simulink model "wtd_wind_profile_ver1"  (R2014b)
settings: Solver=ode3  StartTime=0.0  StopTime=100  FixedStep=0.002  RelTol=1e-3
undefined symbols (not defined in the file): baseSystemPower, complexPower, internalGenVoltage, nodeVoltage, systemFrequency, windSpeedVec, windturbKbParam
libraries: wtd_library_ver1 x11, simulink x1
settings Model: Creator=Jakub  LastModifiedBy=Jakub
settings DataIOCC: SignalLoggingSaveFormat=ModelDataLogs
settings OptimizationCC: ExpressionDepthLimit=2147483647
settings DebuggingCC: UnderspecifiedInitializationDetection=Classic  MergeDetectMultiDrivingBlocksExec=none  FcnCallInpInsideContextMsg=UseLocalSettings  StateNameClashWarn=warning
settings GRTTargetCC: CombineOutputUpdateFcns=off  GRTInterface=on

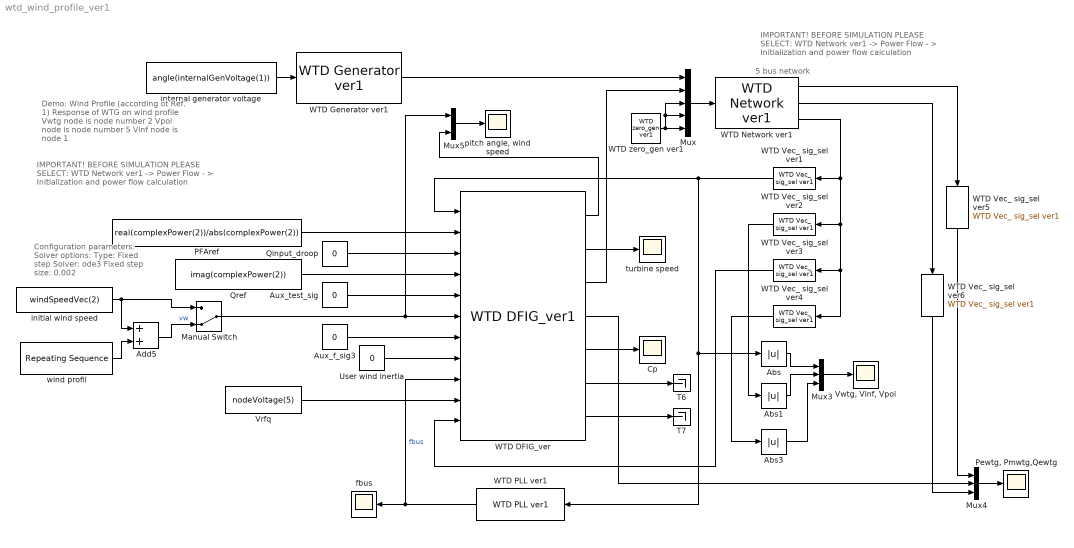
== system wtd_wind_profile_ver1 ==
  note: Demo: Wind Profile
      | (according ot Ref. 1)
      | Response of WTG on wind profile
      | Vwtg node is node number 2
      | Vpoi node is node number 5
      | Vinf node is node 1
  note: IMPORTANT!
      | BEFORE SIMULATION PLEASE SELECT:
      | WTD Network ver1 -> Power Flow - >
      | Initialization and power flow calculation
  note: Configuration parameters:
      | Solver options:
      | Type: Fixed step
      | Solver: ode3
      | Fixed step size: 0.002
  note: 5 bus network
  note: IMPORTANT!
      | BEFORE SIMULATION PLEASE SELECT:
      | WTD Network ver1 -> Power Flow - >
      | Initialization and power flow calculation
  Abs : Abs
  Abs1 : Abs
  Abs3 : Abs
  Add5 : Sum
  Aux_f_sig3 : Constant  Value=0
  Aux_test_sig : Constant  Value=0
  Cp : Scope
      settings: YMin=0.17  YMax=0.24  SaveName=ScopeData13  MaxDataPoints=500000
  Manual Switch : ManualSwitch  CurrentSetting=0
  Mux : Mux  Inputs=5
  Mux3 : Mux  Inputs=3
  Mux4 : Mux  Inputs=3
  Mux5 : Mux  Inputs=2
  PFAref : Constant  Value=real(complexPower(2))/abs(complexPower(2))
  "Pewtg, Pmwtg,Qewtg" : Scope
      settings: YMin=-0.5  YMax=1.5  SaveName=ScopeData3  MaxDataPoints=500000
  Qinput_droop : Constant  Value=0
  Qref : Constant  Value=imag(complexPower(2))
  T6 : Terminator
  T7 : Terminator
  User wind inertia : Constant  Value=0
  Vrfq : Constant  Value=nodeVoltage(5)
  "Vwtg, Vinf, Vpoi" : Scope
      settings: YMin=0.9  YMax=1.1  SaveName=ScopeData9  MaxDataPoints=50000
  WTD Vec_ sig_sel ver6 : wtd_library_ver1/WTD Vec_ sig_sel ver1  SystemSampleTime=-1  node=2
  WTD DFIG_ver : wtd_library_ver1/WTD DFIG_ver1  SystemSampleTime=-1  co_node=2  Sbasesys=baseSystemPower  Sbasem4=100.5  wbase=2*pi*systemFrequency  H=4.94  Xsecsys=genTranReactance  Ka=windturbKaParam  Kb=windturbKbParam  Vwinit=nodeVoltage  Pelec4abs=real(complexPower)*baseSystemPower  Qgen4abs=imag(complexPower)*baseSystemPower  theta=pitchAngleVec  w=turbSpeedVec  pfaflg=0  varflg=1  apcflg=0  Kqd=0  Kpv=18  Kiv=5  Qmax=0.436  Qmin=-0.436  KVi=40  insupp=0  wi_user_GE=0  Kwi=10  Kptrq=3  Kitrq=0.6  Tpc=0.05  dbwi=0.0025  TIpwi=1  Twowi=5.5  urlwi=0.1  drlwi=-1  Pmxwi=0.1  Pmnwi=0
  WTD Generator ver1 : wtd_library_ver1/WTD Generator ver1  SystemSampleTime=-1  co_node=1  E=internalGenVoltage  jxd=genTranReactance
  WTD Network ver1 : wtd_library_ver1/WTD Network ver1  SystemSampleTime=-1  Sbasesys=100  fsystem=60  Ydf=WTD_Y5  no_gen_co=1  no_gen_wi=1  nodes_co=[1]  xd_co=[0.00001]  nodes_wi=2  Pbasemw=100.5  xd_wi=0.8  Ka=0.00159  Kb=56.6  nodes_lo=[]  Sloadabs=[]  flttype=Power  Tfault=inf  nodeadd=3  Saddabs=10  fltimp=0.105  linenumber=1  Tclear=inf  Y2df=WTD_Y5_2  absV_co=1.05  Sgenabs_co=[103,0,85]  wi_choice=Wind_speed  absV_wi=1.007  Sgenabs_wi=60  vw_vector=8.5  pfcalc=off  pffault=on
  WTD PLL ver1 : wtd_library_ver1/WTD PLL ver1  SystemSampleTime=-1  me_node=2  KpPLL=30  KiPLL=0  delta_init_vec=angle(nodeVoltage )  wbase=2*pi*systemFrequency
  WTD Vec_ sig_sel ver1 : wtd_library_ver1/WTD Vec_ sig_sel ver1  SystemSampleTime=-1  node=2
  WTD Vec_ sig_sel ver2 : wtd_library_ver1/WTD Vec_ sig_sel ver1  SystemSampleTime=-1  node=1
  WTD Vec_ sig_sel ver3 : wtd_library_ver1/WTD Vec_ sig_sel ver1  SystemSampleTime=-1  node=5
  WTD Vec_ sig_sel ver4 : wtd_library_ver1/WTD Vec_ sig_sel ver1  SystemSampleTime=-1  node=5
  WTD Vec_ sig_sel ver5 : wtd_library_ver1/WTD Vec_ sig_sel ver1  SystemSampleTime=-1  node=2
  WTD zero_gen ver1 : wtd_library_ver1/WTD zero_gen ver1  SystemSampleTime=-1
  fbus : Scope
      settings: YMin=0.999775  YMax=1.00007  SaveName=ScopeData4  MaxDataPoints=50000
  initial wind speed : Constant  Value=windSpeedVec(2)
  internal generator voltage : Constant  Value=angle(internalGenVoltage(1))
  "pitch angle, wind speed" : Scope
      settings: YMin=0  YMax=20  SaveName=ScopeData5  MaxDataPoints=500000
  turbine speed : Scope
      settings: YMin=0  YMax=1.5  SaveName=ScopeData8  MaxDataPoints=500000
  wind profil : simulink/Sources/Repeating Sequence  rep_seq_t=[0 5 50 62 112 150 190 220 240 350]  rep_seq_y=[0 0 6.235 6.235 -windSpeedVec(2) -windSpeedVec(2) -windSpeedVec(2) -windSpeedVec(2) -windSpeedVec(2) -windSpeedVec(2)]
  wires:
  WTD PLL ver1/1 -> fbus/1, WTD DFIG_ver/9  "fbus"
  Aux_test_sig/1 -> WTD DFIG_ver/5
  Qinput_droop/1 -> WTD DFIG_ver/3
  Qref/1 -> WTD DFIG_ver/4
  PFAref/1 -> WTD DFIG_ver/2
  Manual Switch/1 -> Mux5/1, WTD DFIG_ver/6
  WTD Network ver1/3 -> WTD Vec_ sig_sel ver3/1, WTD Vec_ sig_sel ver4/1, WTD Vec_ sig_sel ver2/1, WTD Vec_ sig_sel ver1/1
  WTD Vec_ sig_sel ver1/1 -> Abs/1, WTD PLL ver1/1, WTD DFIG_ver/1
  WTD Vec_ sig_sel ver2/1 -> Abs1/1
  Mux3/1 -> "Vwtg, Vinf, Vpoi"/1
  Abs/1 -> Mux3/1
  Abs1/1 -> Mux3/2
  Abs3/1 -> Mux3/3
  Mux5/1 -> "pitch angle, wind speed"/1
  Mux4/1 -> "Pewtg, Pmwtg,Qewtg"/1
  Mux/1 -> WTD Network ver1/1
  WTD Generator ver1/1 -> Mux/1
  WTD DFIG_ver/1 -> Mux5/2
  WTD DFIG_ver/2 -> turbine speed/1
  WTD DFIG_ver/5 -> Cp/1
  WTD DFIG_ver/6 -> T6/1
  WTD DFIG_ver/7 -> T7/1
  WTD zero_gen ver1/1 -> Mux/5, Mux/4, Mux/3
  WTD DFIG_ver/4 -> Mux4/2
  WTD Vec_ sig_sel ver4/1 -> Abs3/1
  Aux_f_sig3/1 -> WTD DFIG_ver/7
  WTD DFIG_ver/3 -> Mux/2
  WTD Network ver1/2 -> WTD Vec_ sig_sel ver6/1
  WTD Vec_ sig_sel ver3/1 -> WTD DFIG_ver/11
  Vrfq/1 -> WTD DFIG_ver/10
  User wind inertia/1 -> WTD DFIG_ver/8
  WTD Network ver1/1 -> WTD Vec_ sig_sel ver5/1
  WTD Vec_ sig_sel ver5/1 -> Mux4/1
  WTD Vec_ sig_sel ver6/1 -> Mux4/3
  internal generator voltage/1 -> WTD Generator ver1/1
  initial wind speed/1 -> Add5/1, Manual Switch/1
  wind profil/1 -> Add5/2
  Add5/1 -> Manual Switch/2  "vw"
